simulink model "SF013A_PullCmpActv"  (R2013b)
settings: Solver=FixedStepDiscrete  SolverMode=SingleTasking  StartTime=0.0  StopTime=1  FixedStep=0.002  RelTol=1e-3
values from neighbouring files (symbols this model uses):
  ARCHGLBPRM_100MILLISEC_SEC_F32 = DataDict.Constant    [SF013A_PullCmpActv_DataDict.m]
  ARCHGLBPRM_2MILLISEC_SEC_F32 = DataDict.Constant    [SF013A_PullCmpActv_DataDict.m]
  ARCHGLBPRM_FLOATZEROTHD_ULS_F32 = DataDict.Constant    [SF013A_PullCmpActv_DataDict.m]
  INTGTRSCARSHOTERM_ULS_F32 = DataDict.Constant    [SF013A_PullCmpActv_DataDict.m]
  LONGTERMINTGTRSCAR_ULS_F32 = DataDict.Constant    [SF013A_PullCmpActv_DataDict.m]
  MICROSECTOSEC_ULS_F32 = DataDict.Constant    [SF013A_PullCmpActv_DataDict.m]
  MINSTOSEC_SECPERMINS_F32 = DataDict.Constant    [SF013A_PullCmpActv_DataDict.m]
  PullCmpActvCmpLrnTiDecShoTerm = DataDict.Calibration    [SF013A_PullCmpActv_DataDict.m]
  PullCmpActvCmpLrnTiIncShoTerm = DataDict.Calibration    [SF013A_PullCmpActv_DataDict.m]
  PullCmpActvCmpLrnTiLongTerm = DataDict.Calibration    [SF013A_PullCmpActv_DataDict.m]
  PullCmpActvCmpShoTermRstHwAgThd = DataDict.Calibration    [SF013A_PullCmpActv_DataDict.m]
  PullCmpActvCmpShoTermRstHwTqThd = DataDict.Calibration    [SF013A_PullCmpActv_DataDict.m]
  PullCmpActvCmpShoTermRstLatAThd = DataDict.Calibration    [SF013A_PullCmpActv_DataDict.m]
  PullCmpActvCmpShoTermRstYawRateThd = DataDict.Calibration    [SF013A_PullCmpActv_DataDict.m]
  PullCmpActvEna = DataDict.Calibration    [SF013A_PullCmpActv_DataDict.m]
  PullCmpActvLongTermLim = DataDict.Calibration    [SF013A_PullCmpActv_DataDict.m]
  PullCmpActvLrngEnaAgConfMinMgn = DataDict.Calibration    [SF013A_PullCmpActv_DataDict.m]
  PullCmpActvLrngEnaHwAgMaxMgn = DataDict.Calibration    [SF013A_PullCmpActv_DataDict.m]
  PullCmpActvLrngEnaHwTqMaxMgn = DataDict.Calibration    [SF013A_PullCmpActv_DataDict.m]
  PullCmpActvLrngEnaHwVelMaxMgn = DataDict.Calibration    [SF013A_PullCmpActv_DataDict.m]
  PullCmpActvLrngEnaLatAMaxMgn = DataDict.Calibration    [SF013A_PullCmpActv_DataDict.m]
  PullCmpActvLrngEnaTiThd = DataDict.Calibration    [SF013A_PullCmpActv_DataDict.m]
  PullCmpActvLrngEnaVehSpdMaxMgn = DataDict.Calibration    [SF013A_PullCmpActv_DataDict.m]
  PullCmpActvLrngEnaVehSpdMinMgn = DataDict.Calibration    [SF013A_PullCmpActv_DataDict.m]
  PullCmpActvLrngEnaVehSpdRateMaxMgn = DataDict.Calibration    [SF013A_PullCmpActv_DataDict.m]
  PullCmpActvLrngEnaYawRateMaxMgn = DataDict.Calibration    [SF013A_PullCmpActv_DataDict.m]
  PullCmpActvOpstSignTiShoTerm = DataDict.Calibration    [SF013A_PullCmpActv_DataDict.m]
  PullCmpActvOutpMaxRate = DataDict.Calibration    [SF013A_PullCmpActv_DataDict.m]
  PullCmpActvPullCmpShoTermLim = DataDict.Calibration    [SF013A_PullCmpActv_DataDict.m]
  PullCmpActvPullCmpTotLim = DataDict.Calibration    [SF013A_PullCmpActv_DataDict.m]
  PullCmpActvPullErrLimLongTerm = DataDict.Calibration    [SF013A_PullCmpActv_DataDict.m]
  PullCmpActvPullErrMgnThd = DataDict.Calibration    [SF013A_PullCmpActv_DataDict.m]
  PullCmpActvPullErrShoTermLim = DataDict.Calibration    [SF013A_PullCmpActv_DataDict.m]
  PullCmpActvShoTermRampTi = DataDict.Calibration    [SF013A_PullCmpActv_DataDict.m]
  SysGlbPrmSysTqRat = DataDict.ImprtdCal    [SF013A_PullCmpActv_DataDict.m]
libraries: NxtrAbslt x9, Fil x8, simulink x7, NxtrLim x6, FixdToFloat x3, NxtrSign x3, NxtrMin x3, NxtrNvM x2, NxtrMax x2, FloatToFixd x1, LnrIntrpn x1
(part 1 of 4)
settings Model: Creator=DZVCQL  LastModifiedBy=XZB1DB
settings SolverCC: AutoInsertRateTranBlk=on  InsertRTBMode=Always
settings DataIOCC: LimitDataPoints=off  SaveFormat=Structure  ReturnWorkspaceOutputs=on
settings OptimizationCC: BlockReduction=off  InlineParams=on  ZeroExternalMemoryAtStartup=off  ZeroInternalMemoryAtStartup=off  OptimizeModelRefInitCode=on  LifeSpan=1
settings DebuggingCC: SignalInfNanChecking=error  SignalRangeChecking=warning  ReadBeforeWriteMsg=DisableAll  WriteAfterWriteMsg=DisableAll  WriteAfterReadMsg=DisableAll  UnderspecifiedInitializationDetection=Simplified  SolverPrmCheckMsg=error  InheritedTsInSrcMsg=error  DiscreteInheritContinuousMsg=error  SingleTaskRateTransMsg=error  TasksWithSamePriorityMsg=error  SigSpecEnsureSampleTimeMsg=error  CheckMatrixSingularityMsg=error  ParameterUnderflowMsg=error  ParameterPrecisionLossMsg=error  ParameterTunabilityLossMsg=error  FixptConstUnderflowMsg=warning  FixptConstOverflowMsg=warning  VectorMatrixConversionMsg=error  SignalLabelMismatchMsg=error  UnconnectedInputMsg=error  UnconnectedOutputMsg=error  UnconnectedLineMsg=error  SFcnCompatibilityMsg=error  UniqueDataStoreMsg=warning  BusObjectLabelMismatch=error  RootOutportRequireBusObject=error  AssertControl=DisableAll  ModelReferenceIOMsg=error  ModelReferenceVersionMismatchMessage=warning  ModelReferenceIOMismatchMessage=error  ModelReferenceCSMismatchMessage=warning  ModelReferenceDataLoggingMessage=error  StateNameClashWarn=warning  StrictBusMsg=ErrorOnBusTreatedAsVector  NonBusSignalsTreatedAsBus=error  SFUnexpectedBacktrackingDiag=error  SFInvalidInputDataAccessInChartInitDiag=error  SFNoUnconditionalDefaultTransitionDiag=error  SFTransitionOutsideNaturalParentDiag=error  SFUnconditionalTransitionShadowingDiag=error  SFUndirectedBroadcastEventsDiag=error
settings ModelReferenceCC: ModelReferenceNumInstancesAllowed=Single
settings RTWCC: SystemTargetFile=autosar.tlc  GenCodeOnly=on  TemplateMakefile=ert_default_tmf  Description=AUTOSAR  GenerateReport=on  ProcessScript=autosar_make_rtw_hook  LaunchReport=on
settings CodeAppCC: GenerateComments=off  IgnoreCustomStorageClasses=off  CustomSymbolStrType=$N$R$M  CustomSymbolStrBlkIO=$N$M  SimulinkBlockComments=off
settings STFCustomTargetCC: ParMdlRefBuildCompliant=on  CompOptLevelCompliant=on  IncludeMdlTerminateFcn=off  CombineOutputUpdateFcns=on  SuppressErrorStatus=on  ERTFirstTimeCompliant=on  ERTCustomFileBanners=on  SupportNonFinite=off  SupportComplex=off  SupportContinuousTime=off  SupportNonInlinedSFcns=off  MATLABClassNameForMDSCustomization=Simulink.SoftwareTarget.ERTCustomization  AutosarCompliant=on  GRTInterface=off  SystemTargetFile=autosar.tlc
settings ERTTargetCC: CodeReplacementLibrary=ANSI_C  ConcurrentExecutionCompliant=off  IncludeMdlTerminateFcn=off  SuppressErrorStatus=on  SupportNonFinite=off  SupportComplex=off  ModelStepFunctionPrototypeControlCompliant=off  CPPClassGenCompliant=off  AutosarCompliant=on  InlinedParameterPlacement=NonHierarchical  ERTCustomFileTemplate=example_file_process.tlc  EnableUserReplacementTypes=on

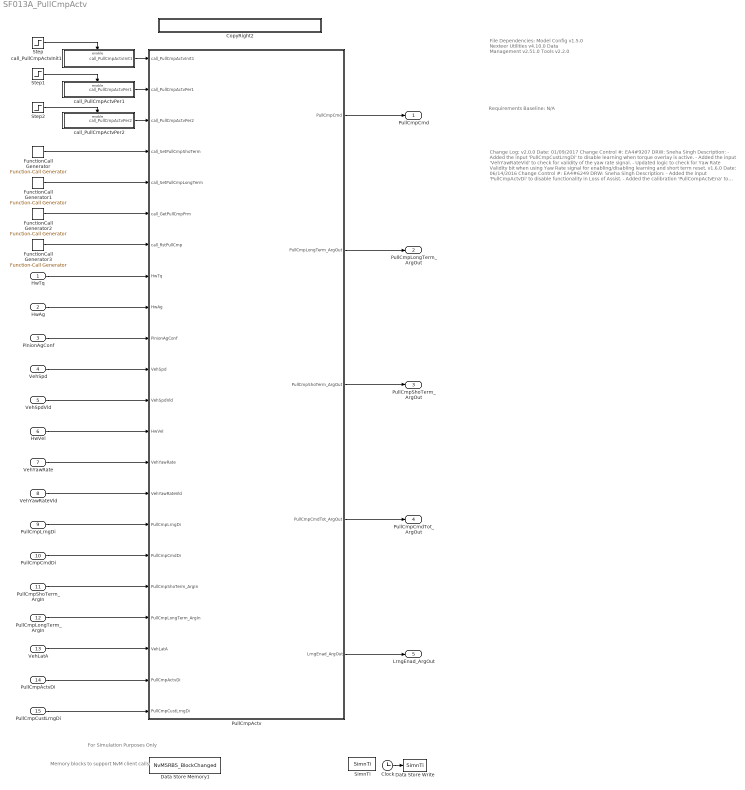
== system SF013A_PullCmpActv ==
  note: Memory blocks to support NvM client calls
  note: For Simulation Purposes Only
  note: File Dependencies:
      |
      | Model Config v1.5.0
      | Nexteer Utilities v4.10.0
      | Data Management v2.51.0
      | Tools v2.2.0
  note: Requirements Baseline: N/A
  note: Change Log:
      |
      | v2.0.0
      | Date: 01/09/2017
      | Change Control #: EA4#9207
      | DRW: Sneha Singh
      | Description:
      | - Added the input 'PullCmpCustLrngDi' to disable learning when torque overlay is active.
      | - Added the input 'VehYawRateVld' to check for validity of the yaw rate signal.
      | - Updated logic to check for Yaw Rate Validity bit when using Yaw Rate signal for
      | enabling/disabling learning and short term reset.
      |
      | v1.6.0
      | Date: 06/14/2016
      | Change Control #: EA4#6249
      | DRW: Sneha Singh
      | Description:
      | - Added the input 'PullCmpActvDi' to disable functionality in Loss of Assist.
      | - Added the calibration 'PullCompActvEna' to execute the function only when the calibration value is True.
      |
      | v1.5.0
      | Date: 03/07/2016
      | Change Control #: EA4#4164
      | DRW:Chang Wang
      | Description:
      | - Corrected ReadIn propertities for input signals PullCmpCmdDi, HwTq and VehSpd in data dictionary.
      |
      |
      | v1.4.0
      | Date: 02/03/2016
      | Change Control #: EA4#3446, EA4#3523
      | DRW:Chang Wang
      | Description:
      | - Removed PullCmpActvCmpShoTermRstYawRate in the data dictionary as duplicated calibration.
      | - Added VehLatA as the new input to the function for the new functionality, enabling  learning and reset
      | short term learning based on lateral acceleration.
      | - Changed min and max value for PIM PullCmpCmdTot.
      | - Enabled StateMustResolveToSignalObject for IntgtrGainIncShoTerm and IntgtrGainDecShoTerm.
      |
      |
      | v1.3.0
      | Date: 10/15/2015
      | Change Control #: EA4#1967
      | DRW: Price Lefler
      | Description:
      | - Fixed DocUnits for RefTiEnaLrng,  RefTiOpstSign and PullCmpActvOpstSignTiShoTerm.
      | - Fixed design error in the calculation of the short term increasing and decreasing integral gains.
      |
      |
      | v1.2.0
      | Date: 10/2/2015
      | Change Control #: EA4#1009
      | DRW: Price Lefler
      | Description:
      | - Removed GetErrorStatus as a client call in the data dictionary.
      |
      | v1.1.0
      | Date: 9/28/2015
      | Change Control #: EA4#1009
      | DRW: Price Lefler
      | Description:
      | - Timer function usage fixed.
      | - ReadIn and WrittenIn properties fixed for the IRV RampDwnStepSize.
      | - Not equal to comparisons for floating point numbers removed and replaced with a difference and
      | a comparison to ARCHGLBPRM_FLOATZEROTHD_ULS_F32
      | - Removed check of GetErrorStatus for PullCmpLongTerm in the model.
      | - Removed the link to undesired requirement.
      |
      | v1.0.0
      | Date:
      | Change Control #: EA4#1009
      | DRW: Chang Wang
      | Description:
      | - Initial Release
      | - Created from EA3 v003
      | - Level 1 model
  HwTq : Inport
  HwAg : Inport  Port=2
  PinionAgConf : Inport  Port=3
  VehSpd : Inport  Port=4
  VehSpdVld : Inport  Port=5
  HwVel : Inport  Port=6
  VehYawRate : Inport  Port=7
  VehYawRateVld : Inport  Port=8
  PullCmpLrngDi : Inport  Port=9
  PullCmpCmdDi : Inport  Port=10
  PullCmpShoTerm_ArgIn : Inport  Port=11
  PullCmpLongTerm_ArgIn : Inport  Port=12
  VehLatA : Inport  Port=13
  PullCmpActvDi : Inport  Port=14
  PullCmpCustLrngDi : Inport  Port=15
  Clock : Clock
  CopyRight2 : Subsystem  Description=|  mask(Copyright Information){none=on}
      | Copyright info block.                                               
      |                                                                     
      | Place copyright information at the top of every subsystem in design.
      mask prompts: none "No parameters"
      mask help: Place copyright information at the top of every subsystem in design.
      mask Display:
      | NxtrConf = 'Nexteer Confidential';
      | 
      | sys = bdroot; %handle for the current model ("system")
      | first = get_param(sys,'Created');
      | if(isempty(first))
      |     first = datestr(now,'yyyy');
      | else
      |     first = first(end-3:end);  %year is last four digits
      | end
      | 
      | last = get_param(sys,'LastModifiedDate');
      | if isempty(last)
      |     last = datestr(now,'yyyy');
      | else
      |     last = last(end-3:end);
      | end
      | 
      | if strcmp(first,last)
      |     fprintf('%s -- Copyright %s Nexteer',NxtrConf,first)
      | else
      |     fprintf('%s -- %s%s- %s Nexteer',NxtrConf,char(169),first,last)
      | end
  Data Store Memory1 : DataStoreMemory  DataStoreName=NvMSRBS_BlockChanged  ReadBeforeWriteMsg=warning  WriteAfterWriteMsg=warning  WriteAfterReadMsg=warning
  Data Store Write : DataStoreWrite  DataStoreName=SimnTi
  FunctionCall Generator{,1..3} (4 alike) : simulink/Ports & Subsystems/Function-Call Generator  sample_time=0.002  numberOfIterations=1
  PullCmpActv : Subsystem
  SimnTi : DataStoreMemory  DataStoreName=SimnTi
  Step : Step  Before=1  After=0  SampleTime=0.002
  Step1 : Step  SampleTime=0.002
  Step2 : Step  SampleTime=0.1
  call_PullCmpActvInit1 : Subsystem  TreatAsAtomicUnit=on
  call_PullCmpActvPer1 : Subsystem  TreatAsAtomicUnit=on
  call_PullCmpActvPer2 : Subsystem  TreatAsAtomicUnit=on
  PullCmpCmd : Outport
  PullCmpLongTerm_ArgOut : Outport  Port=2
  PullCmpShoTerm_ArgOut : Outport  Port=3
  PullCmpCmdTot_ArgOut : Outport  Port=4
  LrngEnad_ArgOut : Outport  Port=5
  wires:
  Clock/1 -> Data Store Write/1
  HwTq/1 -> PullCmpActv/8(HwTq)
  HwAg/1 -> PullCmpActv/9(HwAg)
  PinionAgConf/1 -> PullCmpActv/10(PinionAgConf)
  VehSpd/1 -> PullCmpActv/11(VehSpd)
  VehSpdVld/1 -> PullCmpActv/12(VehSpdVld)
  HwVel/1 -> PullCmpActv/13(HwVel)
  VehYawRate/1 -> PullCmpActv/14(VehYawRate)
  PullCmpLrngDi/1 -> PullCmpActv/16(PullCmpLrngDi)
  PullCmpCmdDi/1 -> PullCmpActv/17(PullCmpCmdDi)
  PullCmpShoTerm_ArgIn/1 -> PullCmpActv/18(PullCmpShoTerm_ArgIn)
  PullCmpActv/1(PullCmpCmd) -> PullCmpCmd/1
  PullCmpActv/2(PullCmpLongTerm_ArgOut) -> PullCmpLongTerm_ArgOut/1
  PullCmpActv/3(PullCmpShoTerm_ArgOut) -> PullCmpShoTerm_ArgOut/1
  PullCmpActv/4(PullCmpCmdTot_ArgOut) -> PullCmpCmdTot_ArgOut/1
  PullCmpActv/5(LrngEnad_ArgOut) -> LrngEnad_ArgOut/1
  VehLatA/1 -> PullCmpActv/20(VehLatA)
  PullCmpActvDi/1 -> PullCmpActv/21(PullCmpActvDi)
  PullCmpCustLrngDi/1 -> PullCmpActv/22(PullCmpCustLrngDi)
  PullCmpLongTerm_ArgIn/1 -> PullCmpActv/19(PullCmpLongTerm_ArgIn)
  call_PullCmpActvInit1/1(call_PullCmpActvInit1) -> PullCmpActv/1(call_PullCmpActvInit1)
  call_PullCmpActvPer1/1(call_PullCmpActvPer1) -> PullCmpActv/2(call_PullCmpActvPer1)
  FunctionCall Generator3/1 -> PullCmpActv/7(call_RstPullCmp)
  VehYawRateVld/1 -> PullCmpActv/15(VehYawRateVld)
  Step/1 -> call_PullCmpActvInit1/Enable
  Step1/1 -> call_PullCmpActvPer1/Enable
  call_PullCmpActvPer2/1(call_PullCmpActvPer2) -> PullCmpActv/3(call_PullCmpActvPer2)
  Step2/1 -> call_PullCmpActvPer2/Enable
  FunctionCall Generator/1 -> PullCmpActv/4(call_SetPullCmpShoTerm)
  FunctionCall Generator1/1 -> PullCmpActv/5(call_SetPullCmpLongTerm)
  FunctionCall Generator2/1 -> PullCmpActv/6(call_GetPullCmpPrm)

== system SF013A_PullCmpActv/CopyRight2 ==

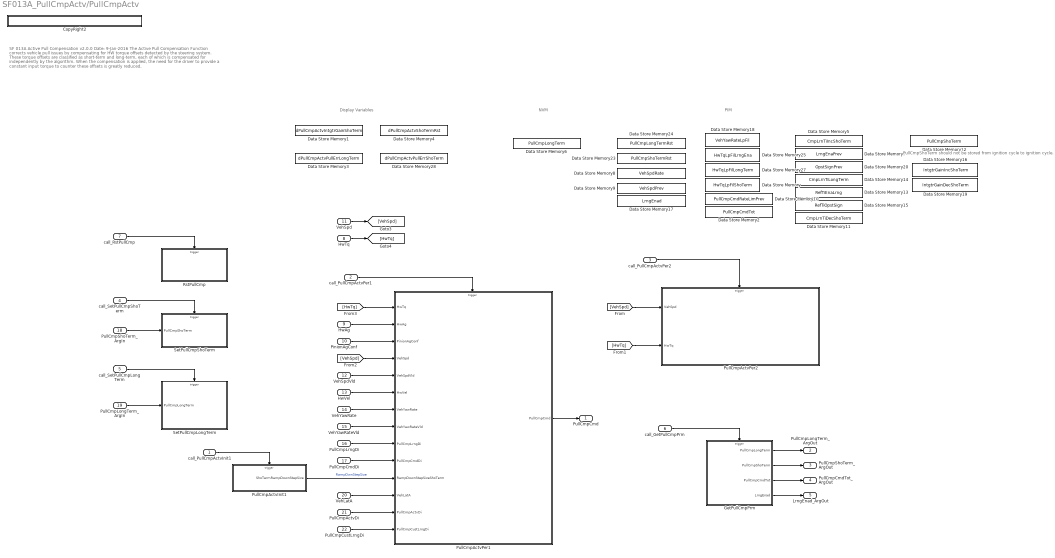
== system SF013A_PullCmpActv/PullCmpActv ==
  note: PullCmpShoTerm should not be stored from ignition cycle to ignition cycle.
  note: Display Variables
  note: SF 013A  Active Pull Compensation
      | v2.0.0      Date: 9-Jan-2016
      |
      | The Active Pull Compensation Function corrects vehicle pull issues by compensating for HW torque offsets detected by the steering system.
      | These torque offsets are classified as short-term and long-term, each of which is compensated for independently by the algorithm.  When
      | the compensation is applied, the need for the driver to provide a constant input torque to counter these offsets is greatly reduced.
  note: NVM
  note: PIM
  call_PullCmpActvInit1 : Inport
  call_PullCmpActvPer1 : Inport  Port=2
  call_PullCmpActvPer2 : Inport  Port=3
  call_SetPullCmpShoTerm : Inport  Port=4
  call_SetPullCmpLongTerm : Inport  Port=5
  call_GetPullCmpPrm : Inport  Port=6
  call_RstPullCmp : Inport  Port=7
  HwTq : Inport  Port=8
  HwAg : Inport  Port=9
  PinionAgConf : Inport  Port=10
  VehSpd : Inport  Port=11
  VehSpdVld : Inport  Port=12
  HwVel : Inport  Port=13
  VehYawRate : Inport  Port=14
  VehYawRateVld : Inport  Port=15
  PullCmpLrngDi : Inport  Port=16
  PullCmpCmdDi : Inport  Port=17
  PullCmpShoTerm_ArgIn : Inport  Port=18
  PullCmpLongTerm_ArgIn : Inport  Port=19
  VehLatA : Inport  Port=20
  PullCmpActvDi : Inport  Port=21
  PullCmpCustLrngDi : Inport  Port=22
  CopyRight2 : Subsystem  Description=|  mask(Copyright Information){none=on}
      | Copyright info block.                                               
      |                                                                     
      | Place copyright information at the top of every subsystem in design.
      mask prompts: none "No parameters"
      mask help: Place copyright information at the top of every subsystem in design.
      mask Display:
      | NxtrConf = 'Nexteer Confidential';
      | 
      | sys = bdroot; %handle for the current model ("system")
      | first = get_param(sys,'Created');
      | if(isempty(first))
      |     first = datestr(now,'yyyy');
      | else
      |     first = first(end-3:end);  %year is last four digits
      | end
      | 
      | last = get_param(sys,'LastModifiedDate');
      | if isempty(last)
      |     last = datestr(now,'yyyy');
      | else
      |     last = last(end-3:end);
      | end
      | 
      | if strcmp(first,last)
      |     fprintf('%s -- Copyright %s Nexteer',NxtrConf,first)
      | else
      |     fprintf('%s -- %s%s- %s Nexteer',NxtrConf,char(169),first,last)
      | end
  Data Store Memory : DataStoreMemory  DataStoreName=HwTqLpFilShoTerm  ReadBeforeWriteMsg=warning  WriteAfterWriteMsg=warning  WriteAfterReadMsg=warning  InitialValue=[]  StateMustResolveToSignalObject=on
  Data Store Memory1 : DataStoreMemory  DataStoreName=dPullCmpActvIntgtrGainShoTerm  ReadBeforeWriteMsg=warning  WriteAfterWriteMsg=warning  WriteAfterReadMsg=warning  StateMustResolveToSignalObject=on
  Data Store Memory10 : DataStoreMemory  DataStoreName=PullCmpCmdRateLimPrev  ReadBeforeWriteMsg=warning  WriteAfterWriteMsg=warning  WriteAfterReadMsg=warning  StateMustResolveToSignalObject=on
  Data Store Memory11 : DataStoreMemory  DataStoreName=CmpLrnTiDecShoTerm  ReadBeforeWriteMsg=warning  WriteAfterWriteMsg=warning  WriteAfterReadMsg=warning  StateMustResolveToSignalObject=on
  Data Store Memory12 : DataStoreMemory  DataStoreName=PullCmpShoTerm  ReadBeforeWriteMsg=warning  WriteAfterWriteMsg=warning  WriteAfterReadMsg=warning  StateMustResolveToSignalObject=on
  Data Store Memory13 : DataStoreMemory  DataStoreName=RefTiEnaLrng  ReadBeforeWriteMsg=warning  WriteAfterWriteMsg=warning  WriteAfterReadMsg=warning  StateMustResolveToSignalObject=on
  Data Store Memory14 : DataStoreMemory  DataStoreName=CmpLrnTiLongTerm  ReadBeforeWriteMsg=warning  WriteAfterWriteMsg=warning  WriteAfterReadMsg=warning  StateMustResolveToSignalObject=on
  Data Store Memory15 : DataStoreMemory  DataStoreName=RefTiOpstSign  ReadBeforeWriteMsg=warning  WriteAfterWriteMsg=warning  WriteAfterReadMsg=warning  StateMustResolveToSignalObject=on
  Data Store Memory16 : DataStoreMemory  DataStoreName=IntgtrGainIncShoTerm  ReadBeforeWriteMsg=warning  WriteAfterWriteMsg=warning  WriteAfterReadMsg=warning  StateMustResolveToSignalObject=on
  Data Store Memory17 : DataStoreMemory  DataStoreName=LrngEnad  ReadBeforeWriteMsg=warning  WriteAfterWriteMsg=warning  WriteAfterReadMsg=warning  StateMustResolveToSignalObject=on
  Data Store Memory18 : DataStoreMemory  DataStoreName=VehYawRateLpFil  ReadBeforeWriteMsg=warning  WriteAfterWriteMsg=warning  WriteAfterReadMsg=warning  InitialValue=[]  StateMustResolveToSignalObject=on
  Data Store Memory19 : DataStoreMemory  DataStoreName=IntgtrGainDecShoTerm  ReadBeforeWriteMsg=warning  WriteAfterWriteMsg=warning  WriteAfterReadMsg=warning  StateMustResolveToSignalObject=on
  Data Store Memory2 : DataStoreMemory  DataStoreName=PullCmpCmdTot  ReadBeforeWriteMsg=warning  WriteAfterWriteMsg=warning  WriteAfterReadMsg=warning  StateMustResolveToSignalObject=on
  Data Store Memory20 : DataStoreMemory  DataStoreName=OpstSignPrev  ReadBeforeWriteMsg=warning  WriteAfterWriteMsg=warning  WriteAfterReadMsg=warning  StateMustResolveToSignalObject=on
  Data Store Memory23 : DataStoreMemory  DataStoreName=PullCmpShoTermRst  ReadBeforeWriteMsg=warning  WriteAfterWriteMsg=warning  WriteAfterReadMsg=warning  StateMustResolveToSignalObject=on
  Data Store Memory24 : DataStoreMemory  DataStoreName=PullCmpLongTermRst  ReadBeforeWriteMsg=warning  WriteAfterWriteMsg=warning  WriteAfterReadMsg=warning  StateMustResolveToSignalObject=on
  Data Store Memory25 : DataStoreMemory  DataStoreName=HwTqLpFilLrngEna  ReadBeforeWriteMsg=warning  WriteAfterWriteMsg=warning  WriteAfterReadMsg=warning  InitialValue=[]  StateMustResolveToSignalObject=on
  Data Store Memory27 : DataStoreMemory  DataStoreName=HwTqLpFilLongTerm  ReadBeforeWriteMsg=warning  WriteAfterWriteMsg=warning  WriteAfterReadMsg=warning  InitialValue=[]  StateMustResolveToSignalObject=on
  Data Store Memory28 : DataStoreMemory  DataStoreName=dPullCmpActvPullErrShoTerm  ReadBeforeWriteMsg=warning  WriteAfterWriteMsg=warning  WriteAfterReadMsg=warning  StateMustResolveToSignalObject=on
  Data Store Memory3 : DataStoreMemory  DataStoreName=dPullCmpActvPullErrLongTerm  ReadBeforeWriteMsg=warning  WriteAfterWriteMsg=warning  WriteAfterReadMsg=warning  StateMustResolveToSignalObject=on
  Data Store Memory4 : DataStoreMemory  DataStoreName=dPullCmpActvShoTermRst  ReadBeforeWriteMsg=warning  WriteAfterWriteMsg=warning  WriteAfterReadMsg=warning  StateMustResolveToSignalObject=on
  Data Store Memory5 : DataStoreMemory  DataStoreName=CmpLrnTiIncShoTerm  ReadBeforeWriteMsg=warning  WriteAfterWriteMsg=warning  WriteAfterReadMsg=warning  StateMustResolveToSignalObject=on
  Data Store Memory6 : DataStoreMemory  DataStoreName=PullCmpLongTerm  ReadBeforeWriteMsg=warning  WriteAfterWriteMsg=warning  WriteAfterReadMsg=warning  StateMustResolveToSignalObject=on
  Data Store Memory7 : DataStoreMemory  DataStoreName=LrngEnaPrev  ReadBeforeWriteMsg=warning  WriteAfterWriteMsg=warning  WriteAfterReadMsg=warning  StateMustResolveToSignalObject=on
  Data Store Memory8 : DataStoreMemory  DataStoreName=VehSpdRate  ReadBeforeWriteMsg=warning  WriteAfterWriteMsg=warning  WriteAfterReadMsg=warning  StateMustResolveToSignalObject=on
  Data Store Memory9 : DataStoreMemory  DataStoreName=VehSpdPrev  ReadBeforeWriteMsg=warning  WriteAfterWriteMsg=warning  WriteAfterReadMsg=warning  StateMustResolveToSignalObject=on
  GetPullCmpPrm : Subsystem  TreatAsAtomicUnit=on
  PullCmpActvInit1 : Subsystem  TreatAsAtomicUnit=on
  PullCmpActvPer1 : Subsystem  TreatAsAtomicUnit=on
  PullCmpActvPer2 : Subsystem  TreatAsAtomicUnit=on
  RstPullCmp : Subsystem  TreatAsAtomicUnit=on
  SetPullCmpLongTerm : Subsystem  TreatAsAtomicUnit=on
  SetPullCmpShoTerm : Subsystem  TreatAsAtomicUnit=on
  PullCmpCmd : Outport
  PullCmpLongTerm_ArgOut : Outport  Port=2
  PullCmpShoTerm_ArgOut : Outport  Port=3
  PullCmpCmdTot_ArgOut : Outport  Port=4
  LrngEnad_ArgOut : Outport  Port=5
  wires:
  GetPullCmpPrm/4(LrngEnad) -> LrngEnad_ArgOut/1
  GetPullCmpPrm/3(PullCmpCmdTot) -> PullCmpCmdTot_ArgOut/1
  GetPullCmpPrm/2(PullCmpShoTerm) -> PullCmpShoTerm_ArgOut/1
  GetPullCmpPrm/1(PullCmpLongTerm) -> PullCmpLongTerm_ArgOut/1
  call_PullCmpActvPer1/1 -> PullCmpActvPer1/Trigger
  call_PullCmpActvInit1/1 -> PullCmpActvInit1/Trigger
  call_PullCmpActvPer2/1 -> PullCmpActvPer2/Trigger
  call_SetPullCmpShoTerm/1 -> SetPullCmpShoTerm/Trigger
  call_SetPullCmpLongTerm/1 -> SetPullCmpLongTerm/Trigger
  call_GetPullCmpPrm/1 -> GetPullCmpPrm/Trigger
  HwTq/1 -> [HwTq]
  HwAg/1 -> PullCmpActvPer1/2("HwAg ")
  PinionAgConf/1 -> PullCmpActvPer1/3("PinionAgConf ")
  VehSpd/1 -> [VehSpd]
  VehSpdVld/1 -> PullCmpActvPer1/5(VehSpdVld)
  HwVel/1 -> PullCmpActvPer1/6(HwVel)
  VehYawRate/1 -> PullCmpActvPer1/7(VehYawRate)
  PullCmpLrngDi/1 -> PullCmpActvPer1/9(PullCmpLrngDi)
  [VehSpd] -> PullCmpActvPer2/1(VehSpd)
  [HwTq] -> PullCmpActvPer2/2(HwTq)
  PullCmpShoTerm_ArgIn/1 -> SetPullCmpShoTerm/1(PullCmpShoTerm)
  PullCmpLongTerm_ArgIn/1 -> SetPullCmpLongTerm/1(PullCmpLongTerm)
  call_RstPullCmp/1 -> RstPullCmp/Trigger
  PullCmpActvPer1/1(PullCmpCmd) -> PullCmpCmd/1
  PullCmpCmdDi/1 -> PullCmpActvPer1/10(PullCmpCmdDi)
  [VehSpd] -> PullCmpActvPer1/4(VehSpd)
  [HwTq] -> PullCmpActvPer1/1(HwTq)
  PullCmpActvInit1/1(ShoTermRampDownStepSize) -> PullCmpActvPer1/11(RampDownStepSizeShoTerm)  "RampDwnStepSize"
  VehLatA/1 -> PullCmpActvPer1/12(VehLatA)
  PullCmpActvDi/1 -> PullCmpActvPer1/13(PullCmpActvDi)
  PullCmpCustLrngDi/1 -> PullCmpActvPer1/14(PullCmpCustLrngDi)
  VehYawRateVld/1 -> PullCmpActvPer1/8(VehYawRateVld)

== system SF013A_PullCmpActv/call_PullCmpActvInit1 ==
  Enable : EnablePort
  CopyRight2 : Subsystem  Description=|  mask(Copyright Information){none=on}
      | Copyright info block.                                               
      |                                                                     
      | Place copyright information at the top of every subsystem in design.
      mask prompts: none "No parameters"
      mask help: Place copyright information at the top of every subsystem in design.
      mask Display:
      | NxtrConf = 'Nexteer Confidential';
      | 
      | sys = bdroot; %handle for the current model ("system")
      | first = get_param(sys,'Created');
      | if(isempty(first))
      |     first = datestr(now,'yyyy');
      | else
      |     first = first(end-3:end);  %year is last four digits
      | end
      | 
      | last = get_param(sys,'LastModifiedDate');
      | if isempty(last)
      |     last = datestr(now,'yyyy');
      | else
      |     last = last(end-3:end);
      | end
      | 
      | if strcmp(first,last)
      |     fprintf('%s -- Copyright %s Nexteer',NxtrConf,first)
      | else
      |     fprintf('%s -- %s%s- %s Nexteer',NxtrConf,char(169),first,last)
      | end
  Function-Call Generator1 : simulink/Ports & Subsystems/Function-Call Generator  sample_time=0.002  numberOfIterations=1
  call_PullCmpActvInit1 : Outport
  wires:
  Function-Call Generator1/1 -> call_PullCmpActvInit1/1

== system SF013A_PullCmpActv/call_PullCmpActvPer1 ==
  Enable : EnablePort
  CopyRight2 : Subsystem  Description=|  mask(Copyright Information){none=on}
      | Copyright info block.                                               
      |                                                                     
      | Place copyright information at the top of every subsystem in design.
      mask prompts: none "No parameters"
      mask help: Place copyright information at the top of every subsystem in design.
      mask Display:
      | NxtrConf = 'Nexteer Confidential';
      | 
      | sys = bdroot; %handle for the current model ("system")
      | first = get_param(sys,'Created');
      | if(isempty(first))
      |     first = datestr(now,'yyyy');
      | else
      |     first = first(end-3:end);  %year is last four digits
      | end
      | 
      | last = get_param(sys,'LastModifiedDate');
      | if isempty(last)
      |     last = datestr(now,'yyyy');
      | else
      |     last = last(end-3:end);
      | end
      | 
      | if strcmp(first,last)
      |     fprintf('%s -- Copyright %s Nexteer',NxtrConf,first)
      | else
      |     fprintf('%s -- %s%s- %s Nexteer',NxtrConf,char(169),first,last)
      | end
  Function-Call Generator1 : simulink/Ports & Subsystems/Function-Call Generator  sample_time=0.002  numberOfIterations=1
  call_PullCmpActvPer1 : Outport
  wires:
  Function-Call Generator1/1 -> call_PullCmpActvPer1/1

== system SF013A_PullCmpActv/call_PullCmpActvPer2 ==
  Enable : EnablePort
  CopyRight2 : Subsystem  Description=|  mask(Copyright Information){none=on}
      | Copyright info block.                                               
      |                                                                     
      | Place copyright information at the top of every subsystem in design.
      mask prompts: none "No parameters"
      mask help: Place copyright information at the top of every subsystem in design.
      mask Display:
      | NxtrConf = 'Nexteer Confidential';
      | 
      | sys = bdroot; %handle for the current model ("system")
      | first = get_param(sys,'Created');
      | if(isempty(first))
      |     first = datestr(now,'yyyy');
      | else
      |     first = first(end-3:end);  %year is last four digits
      | end
      | 
      | last = get_param(sys,'LastModifiedDate');
      | if isempty(last)
      |     last = datestr(now,'yyyy');
      | else
      |     last = last(end-3:end);
      | end
      | 
      | if strcmp(first,last)
      |     fprintf('%s -- Copyright %s Nexteer',NxtrConf,first)
      | else
      |     fprintf('%s -- %s%s- %s Nexteer',NxtrConf,char(169),first,last)
      | end
  Function-Call Generator1 : simulink/Ports & Subsystems/Function-Call Generator  sample_time=0.1  numberOfIterations=1
  call_PullCmpActvPer2 : Outport
  wires:
  Function-Call Generator1/1 -> call_PullCmpActvPer2/1

== system SF013A_PullCmpActv/PullCmpActv/CopyRight2 ==

== system SF013A_PullCmpActv/PullCmpActv/GetPullCmpPrm ==
  function : TriggerPort  TriggerType=function-call
  CopyRight2 : Subsystem  Description=|  mask(Copyright Information){none=on}
      | Copyright info block.                                               
      |                                                                     
      | Place copyright information at the top of every subsystem in design.
      mask prompts: none "No parameters"
      mask help: Place copyright information at the top of every subsystem in design.
      mask Display:
      | NxtrConf = 'Nexteer Confidential';
      | 
      | sys = bdroot; %handle for the current model ("system")
      | first = get_param(sys,'Created');
      | if(isempty(first))
      |     first = datestr(now,'yyyy');
      | else
      |     first = first(end-3:end);  %year is last four digits
      | end
      | 
      | last = get_param(sys,'LastModifiedDate');
      | if isempty(last)
      |     last = datestr(now,'yyyy');
      | else
      |     last = last(end-3:end);
      | end
      | 
      | if strcmp(first,last)
      |     fprintf('%s -- Copyright %s Nexteer',NxtrConf,first)
      | else
      |     fprintf('%s -- %s%s- %s Nexteer',NxtrConf,char(169),first,last)
      | end
  Data Store Read : DataStoreRead  DataStoreName=PullCmpLongTerm
  Data Store Read1 : DataStoreRead  DataStoreName=PullCmpShoTerm
  Data Store Read2 : DataStoreRead  DataStoreName=PullCmpCmdTot
  Data Store Read3 : DataStoreRead  DataStoreName=LrngEnad
  PullCmpLongTerm : Outport
  PullCmpShoTerm : Outport  Port=2
  PullCmpCmdTot : Outport  Port=3
  LrngEnad : Outport  Port=4
  wires:
  Data Store Read/1 -> PullCmpLongTerm/1
  Data Store Read3/1 -> LrngEnad/1
  Data Store Read2/1 -> PullCmpCmdTot/1
  Data Store Read1/1 -> PullCmpShoTerm/1

== system SF013A_PullCmpActv/PullCmpActv/PullCmpActvInit1 ==
  note: Call to GetErrorStatus removed because error handling for NvM block should be taken care of
      | by the NvM Manager as per the Data Dictionary.
  function : TriggerPort  TriggerType=function-call
  Constant1 : Constant  Value=PullCmpActvPullCmpShoTermLim
  Constant3 : Constant  Value=PullCmpActvShoTermRampTi
  Constant4 : Constant  Value=ARCHGLBPRM_2MILLISEC_SEC_F32
  Constant5 : Constant  RequirementInfo={} %GIDa_7dd5e1a6_3745_4149_8da9_62934d4976cf  OutDataTypeStr=single
  CopyRight2 : Subsystem  Description=|  mask(Copyright Information){none=on}
      | Copyright info block.                                               
      |                                                                     
      | Place copyright information at the top of every subsystem in design.
      mask prompts: none "No parameters"
      mask help: Place copyright information at the top of every subsystem in design.
      mask Display:
      | NxtrConf = 'Nexteer Confidential';
      | 
      | sys = bdroot; %handle for the current model ("system")
      | first = get_param(sys,'Created');
      | if(isempty(first))
      |     first = datestr(now,'yyyy');
      | else
      |     first = first(end-3:end);  %year is last four digits
      | end
      | 
      | last = get_param(sys,'LastModifiedDate');
      | if isempty(last)
      |     last = datestr(now,'yyyy');
      | else
      |     last = last(end-3:end);
      | end
      | 
      | if strcmp(first,last)
      |     fprintf('%s -- Copyright %s Nexteer',NxtrConf,first)
      | else
      |     fprintf('%s -- %s%s- %s Nexteer',NxtrConf,char(169),first,last)
      | end
  Divide1 : Product  Inputs=**/
  PullCmpActvHwTqFilLpInit : Fil/FilLpInit  Ic=0  Ts=ARCHGLBPRM_2MILLISEC_SEC_F32  Freq=PullCmpActvHwTqFilFrqLrngEna  StVar=HwTqLpFilLrngEna
  PullCmpActvHwTqLongTermFilLpInit : Fil/FilLpInit  Ic=0  Ts=ARCHGLBPRM_100MILLISEC_SEC_F32  Freq=PullCmpActvHwTqFilFrqLongTerm  StVar=HwTqLpFilLongTerm
  PullCmpActvHwTqShoTermFilLpInit : Fil/FilLpInit  Ic=0  Ts=ARCHGLBPRM_2MILLISEC_SEC_F32  Freq=PullCmpActvHwTqFilFrqShoTerm  StVar=HwTqLpFilShoTerm
  PullCmpActvYawRateFilLpInit : Fil/FilLpInit  Ic=0  Ts=ARCHGLBPRM_2MILLISEC_SEC_F32  Freq=PullCmpActvYawRateFilFrq  StVar=VehYawRateLpFil
  PullCmpLongTerm_SetRamBlockStatus : NxtrNvM/Set Ram Block Status  RequirementInfo={} %GIDa_d378c946_11fa_4093_99df_efb6ba3e3b6f  FuncName=Set Ram Block Status  NvMBlockName=PullCmpLongTerm  VoidFuncRtn=on  BlockChanged_DSN=NvMSRBS_BlockChanged  Return_DSN=NvMSRBS_Return
      settings: AttributesFormatString=%<FuncName>
  ShoTermRampDownStepSize : Outport
  wires:
  Constant4/1 -> Divide1/1
  Constant3/1 -> Divide1/3
  Constant1/1 -> Divide1/2
  Divide1/1 -> ShoTermRampDownStepSize/1
  Constant5/1 -> PullCmpLongTerm_SetRamBlockStatus/1

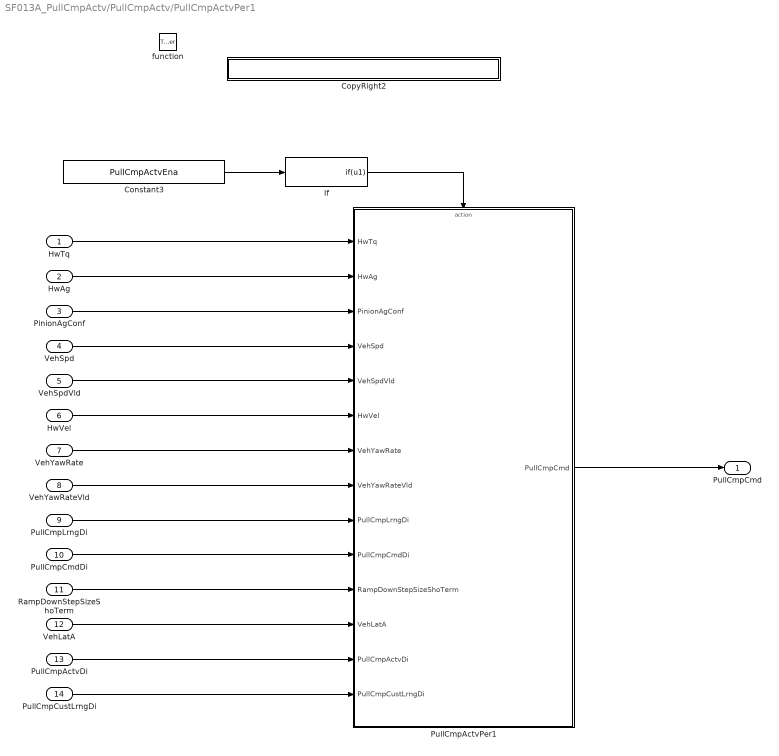
== system SF013A_PullCmpActv/PullCmpActv/PullCmpActvPer1 ==
  HwTq : Inport
  "HwAg " : Inport  Port=2
  "PinionAgConf " : Inport  Port=3
  VehSpd : Inport  Port=4
  VehSpdVld : Inport  Port=5
  HwVel : Inport  Port=6
  VehYawRate : Inport  Port=7
  VehYawRateVld : Inport  Port=8
  PullCmpLrngDi : Inport  Port=9
  PullCmpCmdDi : Inport  Port=10
  RampDownStepSizeShoTerm : Inport  Port=11
  VehLatA : Inport  Port=12
  PullCmpActvDi : Inport  Port=13
  PullCmpCustLrngDi : Inport  Port=14
  function : TriggerPort  TriggerType=function-call
  Constant3 : Constant  Value=PullCmpActvEna
  CopyRight2 : Subsystem  Description=|  mask(Copyright Information){none=on}
      | Copyright info block.                                               
      |                                                                     
      | Place copyright information at the top of every subsystem in design.
      mask prompts: none "No parameters"
      mask help: Place copyright information at the top of every subsystem in design.
      mask Display:
      | NxtrConf = 'Nexteer Confidential';
      | 
      | sys = bdroot; %handle for the current model ("system")
      | first = get_param(sys,'Created');
      | if(isempty(first))
      |     first = datestr(now,'yyyy');
      | else
      |     first = first(end-3:end);  %year is last four digits
      | end
      | 
      | last = get_param(sys,'LastModifiedDate');
      | if isempty(last)
      |     last = datestr(now,'yyyy');
      | else
      |     last = last(end-3:end);
      | end
      | 
      | if strcmp(first,last)
      |     fprintf('%s -- Copyright %s Nexteer',NxtrConf,first)
      | else
      |     fprintf('%s -- %s%s- %s Nexteer',NxtrConf,char(169),first,last)
      | end
  If : If  IfExpression=u1  ShowElse=off
  PullCmpActvPer1 : Subsystem
  PullCmpCmd : Outport
  wires:
  HwTq/1 -> PullCmpActvPer1/1(HwTq)
  "HwAg "/1 -> PullCmpActvPer1/2("HwAg ")
  "PinionAgConf "/1 -> PullCmpActvPer1/3("PinionAgConf ")
  VehSpd/1 -> PullCmpActvPer1/4(VehSpd)
  VehSpdVld/1 -> PullCmpActvPer1/5(VehSpdVld)
  HwVel/1 -> PullCmpActvPer1/6(HwVel)
  VehYawRate/1 -> PullCmpActvPer1/7(VehYawRate)
  PullCmpLrngDi/1 -> PullCmpActvPer1/9(PullCmpLrngDi)
  PullCmpCmdDi/1 -> PullCmpActvPer1/10(PullCmpCmdDi)
  RampDownStepSizeShoTerm/1 -> PullCmpActvPer1/11(RampDownStepSizeShoTerm)
  VehLatA/1 -> PullCmpActvPer1/12(VehLatA)
  PullCmpActvDi/1 -> PullCmpActvPer1/13(PullCmpActvDi)
  PullCmpActvPer1/1(PullCmpCmd) -> PullCmpCmd/1
  If/1 -> PullCmpActvPer1/Action
  Constant3/1 -> If/1
  PullCmpCustLrngDi/1 -> PullCmpActvPer1/14(PullCmpCustLrngDi)
  VehYawRateVld/1 -> PullCmpActvPer1/8(VehYawRateVld)

== system SF013A_PullCmpActv/PullCmpActv/PullCmpActvPer2 ==
  VehSpd : Inport
  HwTq : Inport  Port=2
  function : TriggerPort  TriggerType=function-call
  Constant3 : Constant  Value=PullCmpActvEna
  CopyRight2 : Subsystem  Description=|  mask(Copyright Information){none=on}
      | Copyright info block.                                               
      |                                                                     
      | Place copyright information at the top of every subsystem in design.
      mask prompts: none "No parameters"
      mask help: Place copyright information at the top of every subsystem in design.
      mask Display:
      | NxtrConf = 'Nexteer Confidential';
      | 
      | sys = bdroot; %handle for the current model ("system")
      | first = get_param(sys,'Created');
      | if(isempty(first))
      |     first = datestr(now,'yyyy');
      | else
      |     first = first(end-3:end);  %year is last four digits
      | end
      | 
      | last = get_param(sys,'LastModifiedDate');
      | if isempty(last)
      |     last = datestr(now,'yyyy');
      | else
      |     last = last(end-3:end);
      | end
      | 
      | if strcmp(first,last)
      |     fprintf('%s -- Copyright %s Nexteer',NxtrConf,first)
      | else
      |     fprintf('%s -- %s%s- %s Nexteer',NxtrConf,char(169),first,last)
      | end
  If1 : If  IfExpression=u1  ShowElse=off
  PullCmpActvPer2 : Subsystem
  wires:
  If1/1 -> PullCmpActvPer2/Action
  Constant3/1 -> If1/1
  VehSpd/1 -> PullCmpActvPer2/1(VehSpd)
  HwTq/1 -> PullCmpActvPer2/2(HwTq)

== system SF013A_PullCmpActv/PullCmpActv/RstPullCmp ==
  function : TriggerPort  TriggerType=function-call
  Constant : Constant  OutDataTypeStr=boolean
  Constant1 : Constant  OutDataTypeStr=boolean
  CopyRight2 : Subsystem  Description=|  mask(Copyright Information){none=on}
      | Copyright info block.                                               
      |                                                                     
      | Place copyright information at the top of every subsystem in design.
      mask prompts: none "No parameters"
      mask help: Place copyright information at the top of every subsystem in design.
      mask Display:
      | NxtrConf = 'Nexteer Confidential';
      | 
      | sys = bdroot; %handle for the current model ("system")
      | first = get_param(sys,'Created');
      | if(isempty(first))
      |     first = datestr(now,'yyyy');
      | else
      |     first = first(end-3:end);  %year is last four digits
      | end
      | 
      | last = get_param(sys,'LastModifiedDate');
      | if isempty(last)
      |     last = datestr(now,'yyyy');
      | else
      |     last = last(end-3:end);
      | end
      | 
      | if strcmp(first,last)
      |     fprintf('%s -- Copyright %s Nexteer',NxtrConf,first)
      | else
      |     fprintf('%s -- %s%s- %s Nexteer',NxtrConf,char(169),first,last)
      | end
  Data Store Write : DataStoreWrite  DataStoreName=PullCmpShoTermRst
  Data Store Write1 : DataStoreWrite  DataStoreName=PullCmpLongTermRst
  wires:
  Constant1/1 -> Data Store Write1/1
  Constant/1 -> Data Store Write/1

== system SF013A_PullCmpActv/PullCmpActv/SetPullCmpLongTerm ==
  PullCmpLongTerm : Inport
  function : TriggerPort  TriggerType=function-call
  Constant : Constant  RequirementInfo={} %GIDa_9c81615b_60a0_4dde_9f7a_e3ec35a8c376  OutDataTypeStr=single
  CopyRight2 : Subsystem  Description=|  mask(Copyright Information){none=on}
      | Copyright info block.                                               
      |                                                                     
      | Place copyright information at the top of every subsystem in design.
      mask prompts: none "No parameters"
      mask help: Place copyright information at the top of every subsystem in design.
      mask Display:
      | NxtrConf = 'Nexteer Confidential';
      | 
      | sys = bdroot; %handle for the current model ("system")
      | first = get_param(sys,'Created');
      | if(isempty(first))
      |     first = datestr(now,'yyyy');
      | else
      |     first = first(end-3:end);  %year is last four digits
      | end
      | 
      | last = get_param(sys,'LastModifiedDate');
      | if isempty(last)
      |     last = datestr(now,'yyyy');
      | else
      |     last = last(end-3:end);
      | end
      | 
      | if strcmp(first,last)
      |     fprintf('%s -- Copyright %s Nexteer',NxtrConf,first)
      | else
      |     fprintf('%s -- %s%s- %s Nexteer',NxtrConf,char(169),first,last)
      | end
  Data Store Write : DataStoreWrite  DataStoreName=PullCmpLongTerm
  PullCmpLongTerm_SetRamBlockStatus : NxtrNvM/Set Ram Block Status  RequirementInfo={} %GIDa_05a0e1f5_a949_4242_b915_dab1753a43ae  FuncName=Set Ram Block Status  NvMBlockName=PullCmpLongTerm  VoidFuncRtn=on  BlockChanged_DSN=NvMSRBS_BlockChanged  Return_DSN=NvMSRBS_Return
      settings: AttributesFormatString=%<FuncName>
  wires:
  PullCmpLongTerm/1 -> Data Store Write/1
  Constant/1 -> PullCmpLongTerm_SetRamBlockStatus/1

== system SF013A_PullCmpActv/PullCmpActv/SetPullCmpShoTerm ==
  PullCmpShoTerm : Inport
  function : TriggerPort  TriggerType=function-call
  CopyRight2 : Subsystem  Description=|  mask(Copyright Information){none=on}
      | Copyright info block.                                               
      |                                                                     
      | Place copyright information at the top of every subsystem in design.
      mask prompts: none "No parameters"
      mask help: Place copyright information at the top of every subsystem in design.
      mask Display:
      | NxtrConf = 'Nexteer Confidential';
      | 
      | sys = bdroot; %handle for the current model ("system")
      | first = get_param(sys,'Created');
      | if(isempty(first))
      |     first = datestr(now,'yyyy');
      | else
      |     first = first(end-3:end);  %year is last four digits
      | end
      | 
      | last = get_param(sys,'LastModifiedDate');
      | if isempty(last)
      |     last = datestr(now,'yyyy');
      | else
      |     last = last(end-3:end);
      | end
      | 
      | if strcmp(first,last)
      |     fprintf('%s -- Copyright %s Nexteer',NxtrConf,first)
      | else
      |     fprintf('%s -- %s%s- %s Nexteer',NxtrConf,char(169),first,last)
      | end
  Data Store Write : DataStoreWrite  DataStoreName=PullCmpShoTerm
  wires:
  PullCmpShoTerm/1 -> Data Store Write/1

== system SF013A_PullCmpActv/call_PullCmpActvInit1/CopyRight2 ==

== system SF013A_PullCmpActv/call_PullCmpActvPer1/CopyRight2 ==

== system SF013A_PullCmpActv/call_PullCmpActvPer2/CopyRight2 ==

== system SF013A_PullCmpActv/PullCmpActv/GetPullCmpPrm/CopyRight2 ==

== system SF013A_PullCmpActv/PullCmpActv/PullCmpActvInit1/CopyRight2 ==

== system SF013A_PullCmpActv/PullCmpActv/PullCmpActvPer1/CopyRight2 ==

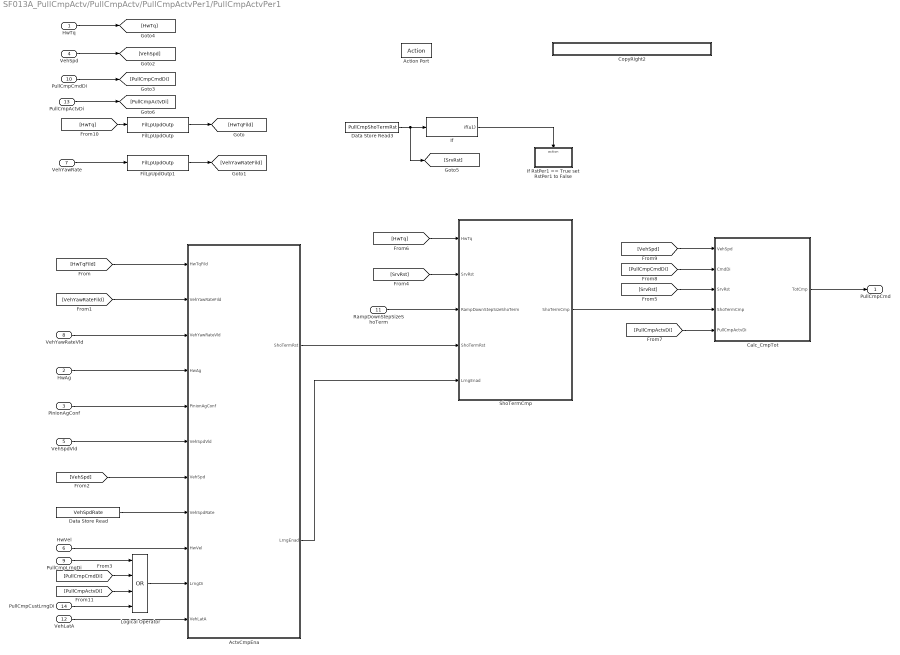
== system SF013A_PullCmpActv/PullCmpActv/PullCmpActvPer1/PullCmpActvPer1 ==
  HwTq : Inport
  "HwAg " : Inport  Port=2
  "PinionAgConf " : Inport  Port=3
  VehSpd : Inport  Port=4
  VehSpdVld : Inport  Port=5
  HwVel : Inport  Port=6
  VehYawRate : Inport  Port=7
  VehYawRateVld : Inport  Port=8
  PullCmpLrngDi : Inport  Port=9
  PullCmpCmdDi : Inport  Port=10
  RampDownStepSizeShoTerm : Inport  Port=11
  VehLatA : Inport  Port=12
  PullCmpActvDi : Inport  Port=13
  PullCmpCustLrngDi : Inport  Port=14
  Action Port : ActionPort  ActionType=then
  ActvCmpEna : Subsystem  TreatAsAtomicUnit=on
  Calc_CmpTot : Subsystem  TreatAsAtomicUnit=on
  CopyRight2 : Subsystem  Description=|  mask(Copyright Information){none=on}
      | Copyright info block.                                               
      |                                                                     
      | Place copyright information at the top of every subsystem in design.
      mask prompts: none "No parameters"
      mask help: Place copyright information at the top of every subsystem in design.
      mask Display:
      | NxtrConf = 'Nexteer Confidential';
      | 
      | sys = bdroot; %handle for the current model ("system")
      | first = get_param(sys,'Created');
      | if(isempty(first))
      |     first = datestr(now,'yyyy');
      | else
      |     first = first(end-3:end);  %year is last four digits
      | end
      | 
      | last = get_param(sys,'LastModifiedDate');
      | if isempty(last)
      |     last = datestr(now,'yyyy');
      | else
      |     last = last(end-3:end);
      | end
      | 
      | if strcmp(first,last)
      |     fprintf('%s -- Copyright %s Nexteer',NxtrConf,first)
      | else
      |     fprintf('%s -- %s%s- %s Nexteer',NxtrConf,char(169),first,last)
      | end
  Data Store Read : DataStoreRead  DataStoreName=VehSpdRate
  Data Store Read3 : DataStoreRead  DataStoreName=PullCmpShoTermRst
  FilLpUpdOutp : Fil/FilLpUpdOutp  StVar=HwTqLpFilLrngEna
      settings: AttributesFormatString=StVar: %<StVar>
  FilLpUpdOutp1 : Fil/FilLpUpdOutp  StVar=VehYawRateLpFil
      settings: AttributesFormatString=StVar: %<StVar>
  If : If  IfExpression=u1  ShowElse=off
  If RstPer1 == True set RstPer1 to False : Subsystem  TreatAsAtomicUnit=on
  Logical Operator : Logic  Operator=OR  Inputs=4  AllPortsSameDT=off  OutDataTypeStr=boolean
  ShoTermCmp : Subsystem  TreatAsAtomicUnit=on
  PullCmpCmd : Outport
  wires:
  HwTq/1 -> [HwTq]
  VehYawRate/1 -> FilLpUpdOutp1/1
  FilLpUpdOutp/1 -> [HwTqFild]
  FilLpUpdOutp1/1 -> [VehYawRateFild]
  [HwTqFild] -> ActvCmpEna/1(HwTqFild)
  [VehYawRateFild] -> ActvCmpEna/2(VehYawRateFild)
  "HwAg "/1 -> ActvCmpEna/4(HwAg)
  "PinionAgConf "/1 -> ActvCmpEna/5(PinionAgConf)
  VehSpdVld/1 -> ActvCmpEna/6(VehSpdVld)
  HwVel/1 -> ActvCmpEna/9(HwVel)
  VehSpd/1 -> [VehSpd]
  [VehSpd] -> ActvCmpEna/7(VehSpd)
  Data Store Read/1 -> ActvCmpEna/8(VehSpdRate)
  PullCmpCmdDi/1 -> [PullCmpCmdDi]
  PullCmpLrngDi/1 -> Logical Operator/1
  Logical Operator/1 -> ActvCmpEna/10(LrngDi)
  [PullCmpCmdDi] -> Logical Operator/2
  [SrvRst] -> ShoTermCmp/2(SrvRst)
  [HwTq] -> ShoTermCmp/1("HwTq ")
  ActvCmpEna/2(LrngEnad) -> ShoTermCmp/5(LrngEnad)
  ShoTermCmp/1(ShoTermCmp) -> Calc_CmpTot/4(ShoTermCmp)
  If/1 -> If RstPer1 == True set RstPer1 to False/Action
  Data Store Read3/1 -> [SrvRst], If/1
  Calc_CmpTot/1(TotCmp) -> PullCmpCmd/1
  [PullCmpCmdDi] -> Calc_CmpTot/2(CmdDi)
  [VehSpd] -> Calc_CmpTot/1(VehSpd)
  [HwTq] -> FilLpUpdOutp/1
  RampDownStepSizeShoTerm/1 -> ShoTermCmp/3(RampDownStepSizeShoTerm)
  [SrvRst] -> Calc_CmpTot/3(SrvRst)
  VehLatA/1 -> ActvCmpEna/11(VehLatA)
  [PullCmpActvDi] -> Calc_CmpTot/5(PullCmpActvDi)
  PullCmpActvDi/1 -> [PullCmpActvDi]
  [PullCmpActvDi] -> Logical Operator/3
  ActvCmpEna/1(ShoTermRst) -> ShoTermCmp/4(ShoTermRst)
  PullCmpCustLrngDi/1 -> Logical Operator/4
  VehYawRateVld/1 -> ActvCmpEna/3(VehYawRateVld)

== system SF013A_PullCmpActv/PullCmpActv/PullCmpActvPer2/CopyRight2 ==

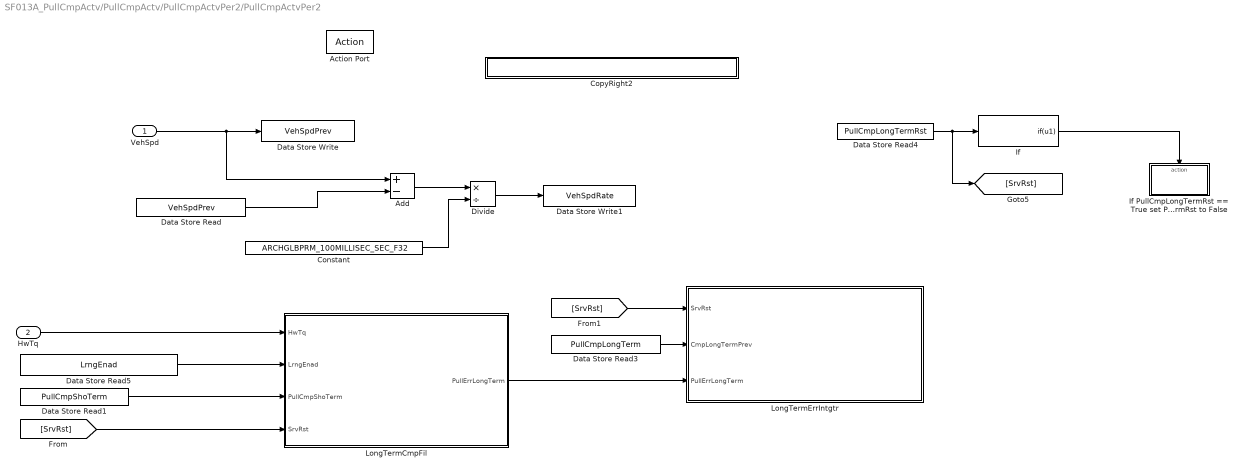
== system SF013A_PullCmpActv/PullCmpActv/PullCmpActvPer2/PullCmpActvPer2 ==
  VehSpd : Inport
  HwTq : Inport  Port=2
  Action Port : ActionPort  ActionType=then
  Add : Sum  Inputs=+-
  Constant : Constant  Value=ARCHGLBPRM_100MILLISEC_SEC_F32
  CopyRight2 : Subsystem  Description=|  mask(Copyright Information){none=on}
      | Copyright info block.                                               
      |                                                                     
      | Place copyright information at the top of every subsystem in design.
      mask prompts: none "No parameters"
      mask help: Place copyright information at the top of every subsystem in design.
      mask Display:
      | NxtrConf = 'Nexteer Confidential';
      | 
      | sys = bdroot; %handle for the current model ("system")
      | first = get_param(sys,'Created');
      | if(isempty(first))
      |     first = datestr(now,'yyyy');
      | else
      |     first = first(end-3:end);  %year is last four digits
      | end
      | 
      | last = get_param(sys,'LastModifiedDate');
      | if isempty(last)
      |     last = datestr(now,'yyyy');
      | else
      |     last = last(end-3:end);
      | end
      | 
      | if strcmp(first,last)
      |     fprintf('%s -- Copyright %s Nexteer',NxtrConf,first)
      | else
      |     fprintf('%s -- %s%s- %s Nexteer',NxtrConf,char(169),first,last)
      | end
  Data Store Read : DataStoreRead  Priority=1  DataStoreName=VehSpdPrev
      settings: AttributesFormatString=priority: %<Priority>
  Data Store Read1 : DataStoreRead  DataStoreName=PullCmpShoTerm
  Data Store Read3 : DataStoreRead  DataStoreName=PullCmpLongTerm
  Data Store Read4 : DataStoreRead  Priority=1  DataStoreName=PullCmpLongTermRst
      settings: AttributesFormatString=priority: %<Priority>
  Data Store Read5 : DataStoreRead  DataStoreName=LrngEnad
  Data Store Write : DataStoreWrite  Priority=2  DataStoreName=VehSpdPrev
      settings: AttributesFormatString=priority: %<Priority>
  Data Store Write1 : DataStoreWrite  DataStoreName=VehSpdRate
  Divide : Product  Inputs=*/
  If : If  IfExpression=u1  ShowElse=off
  If PullCmpLongTermRst == True set PullCmpLongTermRst to False : Subsystem  TreatAsAtomicUnit=on
  LongTermCmpFil : Subsystem  TreatAsAtomicUnit=on
  "LongTermErrIntgtr " : Subsystem  TreatAsAtomicUnit=on
  wires:
  VehSpd/1 -> Add/1, Data Store Write/1
  Data Store Read/1 -> Add/2
  Add/1 -> Divide/1
  Constant/1 -> Divide/2
  Divide/1 -> Data Store Write1/1
  HwTq/1 -> LongTermCmpFil/1("HwTq ")
  [SrvRst] -> LongTermCmpFil/4(SrvRst)
  Data Store Read5/1 -> LongTermCmpFil/2(LrngEnad)
  LongTermCmpFil/1(PullErrLongTerm) -> "LongTermErrIntgtr "/3(PullErrLongTerm)
  Data Store Read3/1 -> "LongTermErrIntgtr "/2(CmpLongTermPrev)
  If/1 -> If PullCmpLongTermRst == True set PullCmpLongTermRst to False/Action
  Data Store Read4/1 -> [SrvRst], If/1
  [SrvRst] -> "LongTermErrIntgtr "/1("SrvRst ")
  Data Store Read1/1 -> LongTermCmpFil/3(PullCmpShoTerm)

== system SF013A_PullCmpActv/PullCmpActv/RstPullCmp/CopyRight2 ==

== system SF013A_PullCmpActv/PullCmpActv/SetPullCmpLongTerm/CopyRight2 ==

== system SF013A_PullCmpActv/PullCmpActv/SetPullCmpShoTerm/CopyRight2 ==
